simulink model "points"  (R2016b)
settings: Solver=FixedStepAuto  StartTime=0.0  StopTime=Inf  RelTol=1e-3  EnableMultiTasking=on
libraries: simulink x6
settings Model: Creator=nmd89  LastModifiedBy=nmd89
settings OptimizationCC: LifeSpan=inf
settings DebuggingCC: SFUnexpectedBacktrackingDiag=warning  SFNoUnconditionalDefaultTransitionDiag=warning  SFExecutionAtInitializationDiag=none
settings GRTTargetCC: TargetLangStandard=C89/C90 (ANSI)  GeneratePreprocessorConditionals=Disable all
settings ConfigComp: CovMetricSettings=dw  CovHtmlReporting=on  CovSaveCumulativeToWorkspaceVar=on  CovSaveSingleToWorkspaceVar=on  CovExternalEMLEnable=off

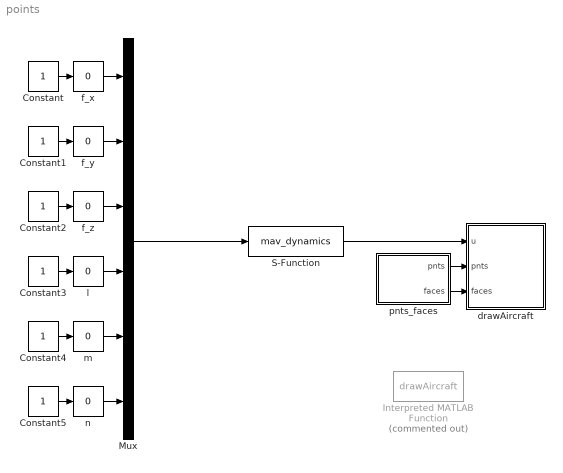
== system points ==
  Constant{,1..5} (6 alike) : Constant
  Interpreted MATLAB Function : MATLABFcn  Commented=on  MATLABFcn=drawAircraft  OutputDimensions=0
      mask init:
      | P.pnts = [...
      |     0.25,     0,       0;
      |     .125,    .1,     -.1;
      |     .125,   -.1,     -.1;
      |     .125,   -.1,      .1;
      |     .125,    .1,      .1;
      |     -.75,      0,      0;
      |        0,     .5,      0;
      |     -.25,     .5,      0;
      |     -.25,    -.5,      0;
      |        0,    -.5,      0;
      |      -.5,    .25,      0;
      |     -.75,    .25,      0;
      |     -.75,   -.25,      0;
      |      -.5,   -.25,      0;
      |      -.5,      0,      0;
      |     -.75,      0,    -.25];
      | 
      | P.faces = [...
      |     1, 2, 3, NaN;
      |     1, 3, 4, NaN;
      |     1, 4, 5, NaN;
      |     1, 2, 5, NaN;
      |     3, 4, 6, NaN;
      |     2, 3, 6, NaN;
      |     2, 5, 6, NaN;
      |     4, 5, 6, NaN;
      |     6, 15, 16, NaN;
      |     11, 12, 13, 14;
      |     7, 8, 9, 10];
  Mux : Mux  Inputs=6
  S-Function : S-Function  FunctionName=mav_dynamics  Parameters=P  SFunctionDeploymentMode=off  EnableBusSupport=off
      mask init:
      | P.pn0 = 0
      | P.pe0 = 0
      | P.pd0 = 0
      | P.u0 = 0
      | P.v0 = 0
      | P.w0 = 0
      | P.phi0 = 0
      | P.th0 = 0
      | P.psi0 = 0
      | P.p0 = 0
      | P.q0 = 0
      | P.r0 = 0
      | P.m = 13.5
      | P.Jx = 0.8244
      | P.Jy = 1.135
      | P.Jz = 1.759
      | P.Jxz = 0.1204
  drawAircraft : MATLAB Function  TreatAsAtomicUnit=on
      mask init:
      | pnts = [...
      |     0.25,     0,       0;
      |     .125,    .1,     -.1;
      |     .125,   -.1,     -.1;
      |     .125,   -.1,      .1;
      |     .125,    .1,      .1;
      |     -.75,      0,      0;
      |        0,     .5,      0;
      |     -.25,     .5,      0;
      |     -.25,    -.5,      0;
      |        0,    -.5,      0;
      |      -.5,    .25,      0;
      |     -.75,    .25,      0;
      |     -.75,   -.25,      0;
      |      -.5,   -.25,      0;
      |      -.5,      0,      0;
      |     -.75,      0,    -.25];
      | 
      | faces = [...
      |     1, 2, 3, NaN;
      |     1, 3, 4, NaN;
      |     1, 4, 5, NaN;
      |     1, 2, 5, NaN;
      |     3, 4, 6, NaN;
      |     2, 3, 6, NaN;
      |     2, 5, 6, NaN;
      |     4, 5, 6, NaN;
      |     6, 15, 16, NaN;
      |     11, 12, 13, 14;
      |     7, 8, 9, 10];
  f_x : simulink/Math Operations/Slider Gain  low=-0.1  gain=0  high=0.1
  f_y : simulink/Math Operations/Slider Gain  low=-0.01  gain=0  high=0.01
  f_z : simulink/Math Operations/Slider Gain  low=-0.01  gain=0  high=0.01
  l : simulink/Math Operations/Slider Gain  low=-0.01  gain=0  high=0.01
  m : simulink/Math Operations/Slider Gain  low=-5  gain=0  high=5
  n : simulink/Math Operations/Slider Gain  low=-5  gain=0  high=5
  pnts_faces : MATLAB Function  TreatAsAtomicUnit=on
  wires:
  f_x/1 -> Mux/1
  f_y/1 -> Mux/2
  f_z/1 -> Mux/3
  l/1 -> Mux/4
  m/1 -> Mux/5
  n/1 -> Mux/6
  Constant/1 -> f_x/1
  Constant1/1 -> f_y/1
  Constant2/1 -> f_z/1
  Constant3/1 -> l/1
  Constant4/1 -> m/1
  Constant5/1 -> n/1
  Mux/1 -> S-Function/1
  S-Function/1 -> drawAircraft/1(u)
  pnts_faces/1(pnts) -> drawAircraft/2(pnts)
  pnts_faces/2(faces) -> drawAircraft/3(faces)

== matlab function points/pnts_faces ==
  data: pnts output; faces output
function [pnts, faces] = pnts_faces

pnts = [...
    0.25,     0,       0;
    .125,    .1,     -.1;
    .125,   -.1,     -.1;
    .125,   -.1,      .1;
    .125,    .1,      .1;
    -.75,      0,      0;
       0,     .5,      0;
    -.25,     .5,      0;
    -.25,    -.5,      0;
       0,    -.5,      0;
     -.5,    .25,      0;
    -.75,    .25,      0;
    -.75,   -.25,      0;
     -.5,   -.25,      0;
     -.5,      0,      0;
    -.75,      0,    -.25];

faces = [...
    1, 2, 3, NaN;
    1, 3, 4, NaN;
    1, 4, 5, NaN;
    1, 2, 5, NaN;
    3, 4, 6, NaN;
    2, 3, 6, NaN;
    2, 5, 6, NaN;
    4, 5, 6, NaN;
    6, 15, 16, NaN;
    11, 12, 13, 14;
    7, 8, 9, 10];

end

== matlab function points/drawAircraft ==
  data: u input; pnts input; faces input
function drawAirCraft(u,pnts,faces)
persistent handle 
coder.extrinsic('patch')

pn = u(1);
pe = u(2);
pd = u(3);
phi = u(7);
tht = u(8);
psi = u(9);

% rotate the aircraft
pnts = rotate(pnts',phi,tht,psi);

% translate the aircraft
pnts = translate(pnts',pn,pe,pd);

% transform vertices from NED to XYZ
R = [...
    0,1,0;
    1,0,0;
    0,0,-1];

pnts = R*pnts';

if isempty(handle)
   handle = patch('Vertices',pnts','Faces',faces,'FaceColor','b');
   axis([-5,5,-5,5,-5,5]);
   grid on
else
   set(handle,'Vertices',pnts','Faces',faces);
%    axis([pn-1,pn+1,pe-1,pe+1,pd-1,pd+1]);
end
